simulink model "AVR_Fuzzy"  (R2020a)
settings: Solver=VariableStepAuto  StartTime=0.0  StopTime=10.0  RelTol=1e-3
libraries: fuzblock x1, simulink x1
settings Model: Creator=Reaga  LastModifiedBy=Reaga

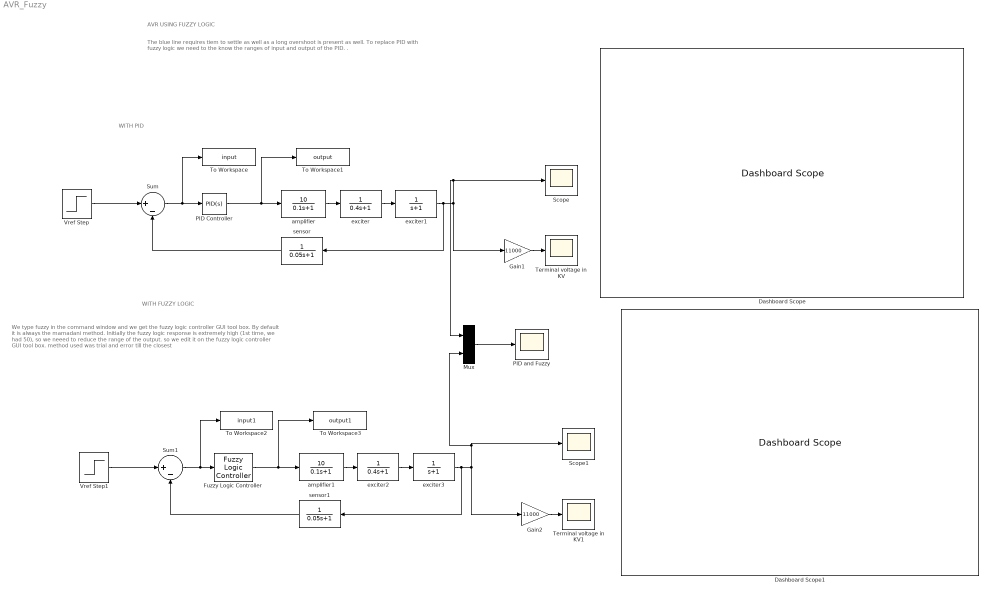
== system AVR_Fuzzy ==
  note: We type fuzzy in the command window and we get the fuzzy logic controller GUI tool box. By default it is always the mamadani method.
      | Initially the fuzzy logic response is extremely high (1st time, we had 50), so we neeed to reduce the range of the output. so we edit it on the fuzzy logic controller GUI tool
      | box.
      | method used was trial and error till the closest
  note: WITH FUZZY LOGIC
  note: WITH PID
  note: The blue line requires tiem to settle as well as a long overshoot is present as well.
      |
      | To replace PID with fuzzy logic we need to the know the ranges of input and output of the PID.
      |
      | .
  note: AVR USING FUZZY LOGIC
  Dashboard Scope : DashboardScope
  Dashboard Scope1 : DashboardScope
  Fuzzy Logic Controller : fuzblock/Fuzzy Logic  Controller  FIS=avr_fuzzy  OutputSampleNumber=101  DataType=double  FuzzifiedInputs=off  RuleFiringStrengths=off  RuleOutputs=off  AggregatedOutputs=off  SimulateUsing=Interpreted execution  OutOfRangeInputValueMessage=warning  NoRuleFiredMessage=warning  EmptyOutputFuzzySetMessage=warning
  Gain1 : Gain  Gain=11000
  Gain2 : Gain  Gain=11000
  Mux : Mux  Inputs=2
  PID Controller : simulink/Continuous/PID Controller  Controller=PID  Form=Parallel  TimeDomain=Continuous-time  UseExternalTs=off  SampleTime=-1  IntegratorMethod=Forward Euler  FilterMethod=Forward Euler  ControllerParametersSource=internal  P=0.21444  I=0.15779  D=0.07058  UseFilter=on  N=100  TunerSelectOption=Transfer Function Based (PID Tuner App)  InitialConditionSource=internal  InitialConditionForIntegrator=0  InitialConditionForFilter=0  DifferentiatorICPrevScaledInput=0  ExternalReset=none  TrackingMode=off  Kt=1  LimitOutput=off  UpperSaturationLimit=inf  LowerSaturationLimit=-inf  LinearizeAsGain=on  AntiWindupMode=none  Kb=1  POutMin=[]  POutMax=[]  IOutMin=[]  IOutMax=[]  DOutMin=[]  DOutMax=[]  NOutMin=[]  NOutMax=[]  SumOutMin=[]  SumOutMax=[]  SaturationOutMin=[]  SaturationOutMax=[]  PParamMin=[]  PParamMax=[]  IParamMin=[]  IParamMax=[]  DParamMin=[]  DParamMax=[]  NParamMin=[]  NParamMax=[]  KbParamMin=[]  KbParamMax=[]  KtParamMin=[]  KtParamMax=[]  KbOutMin=[]  KbOutMax=[]  KtOutMin=[]  KtOutMax=[]  IntegratorOutMin=[]  IntegratorOutMax=[]  FilterOutMin=[]  FilterOutMax=[]  SumI1OutMin=[]  SumI1OutMax=[]  SumI2OutMin=[]  SumI2OutMax=[]  SumI3OutMin=[]  SumI3OutMax=[]  SumI4OutMin=[]  SumI4OutMax=[]  SumDOutMin=[]  SumDOutMax=[]  DifferentiatorOutMin=[]  DifferentiatorOutMax=[]  FilterDiffOutCoefMin=[]  FilterDiffOutCoefMax=[]  ReciprocalOutMin=[]  ReciprocalOutMax=[]  SumDenOutMin=[]  SumDenOutMax=[]  SumNumOutMin=[]  SumNumOutMax=[]  DivideOutMin=[]  DivideOutMax=[]  UdiffTsProdOutMin=[]  UdiffTsProdOutMax=[]  NTsProdOutMin=[]  NTsProdOutMax=[]  UintegralTsProdOutMin=[]  UintegralTsProdOutMax=[]  UngainTsProdOutMin=[]  UngainTsProdOutMax=[]  IntegratorContinuousStateAttributes=''  IntegratorStateMustResolveToSignalObject=off  IntegratorRTWStateStorageClass=Auto  FilterContinuousStateAttributes=''  FilterStateMustResolveToSignalObject=off  FilterRTWStateStorageClass=Auto  ParallelPVariant=InternalParameters  IdealPVariant=Disabled  IVariant=InternalParameters  DVariant=InternalParameters  IntegratorVariant=Continuous  SatVariant=Disabled  AWVariant=Passthrough  PCopyVariant=Disabled  TRVariant=Disabled  FdbkBlocksVariant=Forward  IdealPFdbkVariant=Disabled  SatFdbkVariant=Disabled  DerivativeFilterVariant=ContFilter  NVariant=InternalParameters  NCopyVariant=Disabled  FilterICVariant=InternalICsFilter  IntegratorICVariant=InternalICs  ExternalResetVariant=Disabled  TRSumVariant=Passthrough  SumFdbkVariant=Disabled  SumVariant=Sum_PID  TsampFilterVariant=InternalTs  TsampNgainVariant=Passthrough  TsampIntegralVariant=Passthrough
  PID and Fuzzy : Scope
  Scope : Scope
  Scope1 : Scope
  Sum : Sum  Inputs=|+-
  Sum1 : Sum  Inputs=|+-
  Terminal voltage in KV : Scope
  Terminal voltage in KV1 : Scope
  To Workspace : ToWorkspace  VariableName=input  SaveFormat=Timeseries  SampleTime=-1
  To Workspace1 : ToWorkspace  VariableName=output  SaveFormat=Timeseries  SampleTime=-1
  To Workspace2 : ToWorkspace  VariableName=input1  SaveFormat=Timeseries  SampleTime=-1
  To Workspace3 : ToWorkspace  VariableName=output1  SaveFormat=Timeseries  SampleTime=-1
  Vref Step : Step  Time=20  Before=1  SampleTime=0
  Vref Step1 : Step  Time=20  Before=1  SampleTime=0
  amplifier : TransferFcn  Numerator=[10]  Denominator=[0.1 1]
  amplifier1 : TransferFcn  Numerator=[10]  Denominator=[0.1 1]
  exciter : TransferFcn  Denominator=[0.4 1]
  exciter1 : TransferFcn  Denominator=[1 1]
  exciter2 : TransferFcn  Denominator=[0.4 1]
  exciter3 : TransferFcn  Denominator=[1 1]
  sensor : TransferFcn  Denominator=[0.05 1]
  sensor1 : TransferFcn  Denominator=[0.05 1]
  wires:
  Gain1/1 -> Terminal voltage in KV/1
  Sum/1 -> To Workspace/1, PID Controller/1
  amplifier/1 -> exciter/1
  PID Controller/1 -> To Workspace1/1, amplifier/1
  exciter/1 -> exciter1/1
  Vref Step/1 -> Sum/1
  sensor/1 -> Sum/2
  exciter1/1 -> sensor/1, Gain1/1, Scope/1, Mux/1
  exciter2/1 -> exciter3/1
  amplifier1/1 -> exciter2/1
  sensor1/1 -> Sum1/2
  Sum1/1 -> Fuzzy Logic Controller/1, To Workspace2/1
  Gain2/1 -> Terminal voltage in KV1/1
  Vref Step1/1 -> Sum1/1
  Fuzzy Logic Controller/1 -> To Workspace3/1, amplifier1/1
  exciter3/1 -> sensor1/1, Gain2/1, Mux/2, Scope1/1
  Mux/1 -> PID and Fuzzy/1
